simulink library "rewardLibrary"  (R2022b)
settings: Solver=VariableStepAuto  StartTime=0.0  StopTime=10.0  RelTol=1e-3
values from neighbouring files (symbols this model uses):
  accel_vec = (-4:0.5:4)'    [setUpModel.m]
  Ts = 0.1    [setUpMPC.m]
  TsRL = Ts    [setUpRLEnv.m]
  vel_vec = 0:2:20    [setUpModel.m]
undefined symbols (not defined in the file or in its folder): A, B, C, curvature1, D, D_default, DiscIntNeverNeededParam, E, F, gradbp1, k_sigmoid, steer_lim, t_gap, v_set, x_colpen, y_colpen, Z_colpen
libraries: simulink x379, $bdroot x2, mpcadaslib x1
(part 2 of 9)

== system rewardLibrary/Obs // Reward 6-1 ==
  xgap : Inport
  ygap : Inport  Port=2
  v_lead : Inport  Port=3
  v_ego : Inport  Port=4
  v_ref : Inport  Port=5
  e1 : Inport  Port=6
  e2 : Inport  Port=7
  e1dot : Inport  Port=8
  e2dot : Inport  Port=9
  accel : Inport  Port=10
  steer : Inport  Port=11
  collided : Inport  Port=12
  Abs : Abs  SaturateOnIntegerOverflow=off
  Compare To Constant : simulink/Logic and Bit Operations/Compare To Constant  relop=<=  const=6  OutDataTypeStr=boolean
  Gain1 : Gain  Gain=20
  Gain2 : Gain  Gain=1500
  Logical Operator1 : Logic  Operator=OR  AllPortsSameDT=off  OutDataTypeStr=boolean
  Subsystem : Subsystem
  Subsystem1 : Subsystem
  Subsystem2 : Subsystem
  Sum : Sum  Inputs=-++
  Terminator3 : Terminator
  obs : Outport  VectorParamsAs1DForOutWhenUnconnected=off
  Reward : Outport  Port=2  VectorParamsAs1DForOutWhenUnconnected=off
  isDone : Outport  Port=3  VectorParamsAs1DForOutWhenUnconnected=off
  tag scope: onTrack=global
  wires:
  Gain2/1 -> Sum/2
  Subsystem2/2(success) -> Gain2/1, Logical Operator1/2
  Subsystem2/1(fail) -> Logical Operator1/1, Gain1/1
  v_ego/1 -> Subsystem/1(v_ego), Subsystem2/1(v_ego)
  Logical Operator1/1 -> isDone/1
  accel/1 -> Subsystem1/5(accel)
  steer/1 -> Subsystem1/4(steer)
  Subsystem/2(v_err) -> Subsystem1/1(v_err)
  Subsystem1/1(reward) -> Sum/3
  ygap/1 -> Subsystem/9(ygap)
  v_ref/1 -> Subsystem/2(v_ref)
  collided/1 -> Terminator3/1
  Compare To Constant/1 -> [onTrack]
  Abs/1 -> Compare To Constant/1
  Gain1/1 -> Sum/1
  Sum/1 -> Reward/1
  e1dot/1 -> Subsystem/5(e1dot)
  Subsystem/1(obs) -> obs/1
  xgap/1 -> Subsystem/8(xgap)
  v_lead/1 -> Subsystem/7(v_lead)
  e2/1 -> Subsystem2/3(e2), Subsystem1/3(e2), Subsystem/4(e2)
  e1/1 -> Subsystem2/2(e1), Subsystem/3(e1), Subsystem1/2(e1), Abs/1
  e2dot/1 -> Subsystem/6(e2dot)

== system rewardLibrary/Obs // Reward 6-2 ==
  xgap : Inport
  ygap : Inport  Port=2
  v_lead : Inport  Port=3
  v_ego : Inport  Port=4
  v_ref : Inport  Port=5
  e1 : Inport  Port=6
  e2 : Inport  Port=7
  e1dot : Inport  Port=8
  e2dot : Inport  Port=9
  accel : Inport  Port=10
  steer : Inport  Port=11
  collided : Inport  Port=12
  A : Gain  Gain=1500
  Abs : Abs  SaturateOnIntegerOverflow=off
  B : Gain  Gain=2000
  Compare To Constant : simulink/Logic and Bit Operations/Compare To Constant  relop=<=  const=6  OutDataTypeStr=boolean
  E : Gain  Gain=2000
  Gain1 : Gain  Gain=20
  Logical Operator1 : Logic  Operator=OR  Inputs=3  AllPortsSameDT=off  OutDataTypeStr=boolean
  Overtaking : Subsystem
  Path following : Subsystem
  Subsystem : Subsystem
  Subsystem2 : Subsystem
  Sum : Sum  Inputs=--+++++
  Zone collision penalty : Lookup_n-D  BreakpointsForDimension1=y_colpen  BreakpointsForDimension2=x_colpen  Table=Z_colpen  ExtrapMethod=Clip  InternalRulePriority=Speed  RndMeth=Simplest
      settings: InputPortMap=u0,u1
      mask Display:
      | image("LookupTable.PNG")
      | port_label('input', 1, 'y')
      | port_label('input', 2, 'x')
      | port_label('output', 1, 'p_col')
  obs : Outport  VectorParamsAs1DForOutWhenUnconnected=off
  Reward : Outport  Port=2  VectorParamsAs1DForOutWhenUnconnected=off
  isDone : Outport  Port=3  VectorParamsAs1DForOutWhenUnconnected=off
  tag scope: onTrack=global, p_col=global
  wires:
  A/1 -> Sum/3
  Subsystem2/3(completeCourse) -> Logical Operator1/3, A/1
  Subsystem2/1(fail) -> Gain1/1, Logical Operator1/1
  v_ego/1 -> Subsystem/1(v_ego), Subsystem2/1(v_ego)
  Logical Operator1/1 -> isDone/1
  accel/1 -> Path following/5(accel)
  steer/1 -> Path following/4(steer)
  Subsystem/2(v_err) -> Path following/1(v_err)
  ygap/1 -> Zone collision penalty/1, Subsystem/9(ygap)
  v_ref/1 -> Subsystem/2(v_ref)
  collided/1 -> Subsystem2/5(collided)
  Compare To Constant/1 -> [onTrack]
  Abs/1 -> Compare To Constant/1
  Gain1/1 -> Sum/1
  Sum/1 -> Reward/1
  e1dot/1 -> Subsystem/5(e1dot)
  Subsystem/1(obs) -> obs/1
  xgap/1 -> Overtaking/2(G), Zone collision penalty/2, Subsystem2/4(xgap), Subsystem/8(xgap)
  v_lead/1 -> Subsystem/7(v_lead)
  e2/1 -> Subsystem2/3(e2), Path following/3(e2), Subsystem/4(e2)
  e1/1 -> Subsystem2/2(e1), Subsystem/3(e1), Path following/2(e1), Abs/1
  e2dot/1 -> Subsystem/6(e2dot)
  Path following/1(r_pf) -> Sum/5
  [ry2] -> Overtaking/1(ry)
  Subsystem2/4(overtakeSuccess) -> B/1
  B/1 -> Sum/4
  Overtaking/1(r_ot) -> Sum/6
  Subsystem2/2(failCollided) -> E/1, Logical Operator1/2
  E/1 -> Sum/2
  Zone collision penalty/1 -> Sum/7, [p_col]

== system rewardLibrary/Obs // Reward 6-3 ==
  xgap : Inport
  ygap : Inport  Port=2
  v_lead : Inport  Port=3
  v_ego : Inport  Port=4
  v_ref : Inport  Port=5
  e1 : Inport  Port=6
  e2 : Inport  Port=7
  e1dot : Inport  Port=8
  e2dot : Inport  Port=9
  accel : Inport  Port=10
  steer : Inport  Port=11
  collided : Inport  Port=12
  Abs : Abs  SaturateOnIntegerOverflow=off
  Compare To Constant : simulink/Logic and Bit Operations/Compare To Constant  relop=<=  const=6  OutDataTypeStr=boolean
  Gain1 : Gain  Gain=20
  Gain2 : Gain  Gain=1500
  Gain3 : Gain  Gain=100
  Logical Operator1 : Logic  Operator=OR  Inputs=3  AllPortsSameDT=off  OutDataTypeStr=boolean
  Subsystem : Subsystem
  Subsystem1 : Subsystem
  Subsystem2 : Subsystem
  Sum : Sum  Inputs=--++
  Terminator3 : Terminator
  obs : Outport  VectorParamsAs1DForOutWhenUnconnected=off
  Reward : Outport  Port=2  VectorParamsAs1DForOutWhenUnconnected=off
  isDone : Outport  Port=3  VectorParamsAs1DForOutWhenUnconnected=off
  tag scope: onTrack=global
  wires:
  Gain2/1 -> Sum/3
  Subsystem2/2(success) -> Gain2/1, Logical Operator1/2
  Subsystem2/1(fail) -> Gain1/1, Logical Operator1/1
  v_ego/1 -> Subsystem/1(v_ego), Subsystem2/1(v_ego)
  Logical Operator1/1 -> isDone/1
  accel/1 -> Subsystem1/5(accel)
  steer/1 -> Subsystem1/4(steer)
  Subsystem/2(v_err) -> Subsystem1/1(v_err)
  Subsystem1/1(reward) -> Sum/4
  ygap/1 -> Subsystem/9(ygap)
  v_ref/1 -> Subsystem/2(v_ref)
  collided/1 -> Terminator3/1
  Compare To Constant/1 -> [onTrack]
  Abs/1 -> Compare To Constant/1
  Gain1/1 -> Sum/1
  Sum/1 -> Reward/1
  e1dot/1 -> Subsystem/5(e1dot)
  Subsystem/1(obs) -> obs/1
  xgap/1 -> Subsystem/8(xgap)
  v_lead/1 -> Subsystem/7(v_lead)
  e2/1 -> Subsystem2/3(e2), Subsystem1/3(e2), Subsystem/4(e2)
  e1/1 -> Subsystem2/2(e1), Subsystem/3(e1), Subsystem1/2(e1), Abs/1
  e2dot/1 -> Subsystem/6(e2dot)
  Subsystem2/3(fail_spinTurn) -> Gain3/1, Logical Operator1/3
  Gain3/1 -> Sum/2

== system rewardLibrary/Obs // Reward 6-4 ==
  xgap : Inport
  ygap : Inport  Port=2
  v_lead : Inport  Port=3
  v_ego : Inport  Port=4
  v_ref : Inport  Port=5
  e1 : Inport  Port=6
  e2 : Inport  Port=7
  e1dot : Inport  Port=8
  e2dot : Inport  Port=9
  accel : Inport  Port=10
  steer : Inport  Port=11
  collided : Inport  Port=12
  Abs : Abs  SaturateOnIntegerOverflow=off
  Compare To Constant : simulink/Logic and Bit Operations/Compare To Constant  relop=<=  const=6  OutDataTypeStr=boolean
  Gain1 : Gain  Gain=20
  Gain2 : Gain  Gain=1500
  Logical Operator1 : Logic  Operator=OR  AllPortsSameDT=off  OutDataTypeStr=boolean
  Subsystem : Subsystem
  Subsystem1 : Subsystem
  Subsystem2 : Subsystem
  Sum : Sum  Inputs=-++
  Terminator3 : Terminator
  obs : Outport  VectorParamsAs1DForOutWhenUnconnected=off
  Reward : Outport  Port=2  VectorParamsAs1DForOutWhenUnconnected=off
  isDone : Outport  Port=3  VectorParamsAs1DForOutWhenUnconnected=off
  tag scope: onTrack=global
  wires:
  Gain2/1 -> Sum/2
  Subsystem2/2(success) -> Gain2/1, Logical Operator1/2
  Subsystem2/1(fail) -> Logical Operator1/1, Gain1/1
  v_ego/1 -> Subsystem/1(v_ego), Subsystem2/1(v_ego)
  Logical Operator1/1 -> isDone/1
  accel/1 -> Subsystem1/5(accel)
  steer/1 -> Subsystem1/4(steer)
  Subsystem/2(v_err) -> Subsystem1/1(v_err)
  ygap/1 -> Subsystem/9(ygap)
  v_ref/1 -> Subsystem/2(v_ref)
  collided/1 -> Terminator3/1
  Compare To Constant/1 -> [onTrack]
  Abs/1 -> Compare To Constant/1
  Gain1/1 -> Sum/1
  Sum/1 -> Reward/1
  e1dot/1 -> Subsystem/5(e1dot)
  Subsystem/1(obs) -> obs/1
  xgap/1 -> Subsystem/8(xgap)
  v_lead/1 -> Subsystem/7(v_lead)
  e2/1 -> Subsystem2/3(e2), Subsystem1/3(e2), Subsystem/4(e2)
  e1/1 -> Subsystem2/2(e1), Subsystem/3(e1), Subsystem1/2(e1), Abs/1
  e2dot/1 -> Subsystem/6(e2dot)
  Subsystem1/1(reward) -> Sum/3

== system rewardLibrary/Obs // Reward 6-5 ==
  xgap : Inport
  ygap : Inport  Port=2
  v_lead : Inport  Port=3
  v_ego : Inport  Port=4
  v_ref : Inport  Port=5
  e1 : Inport  Port=6
  e2 : Inport  Port=7
  e1dot : Inport  Port=8
  e2dot : Inport  Port=9
  accel : Inport  Port=10
  steer : Inport  Port=11
  collided : Inport  Port=12
  Abs : Abs  SaturateOnIntegerOverflow=off
  Compare To Constant : simulink/Logic and Bit Operations/Compare To Constant  relop=<=  const=6  OutDataTypeStr=boolean
  Gain1 : Gain  Gain=20
  Gain2 : Gain  Gain=1500
  Logical Operator1 : Logic  Operator=OR  AllPortsSameDT=off  OutDataTypeStr=boolean
  Subsystem : Subsystem
  Subsystem1 : Subsystem
  Subsystem2 : Subsystem
  Sum : Sum  Inputs=-++
  Terminator3 : Terminator
  obs : Outport  VectorParamsAs1DForOutWhenUnconnected=off
  Reward : Outport  Port=2  VectorParamsAs1DForOutWhenUnconnected=off
  isDone : Outport  Port=3  VectorParamsAs1DForOutWhenUnconnected=off
  tag scope: onTrack=global
  wires:
  Gain2/1 -> Sum/2
  Subsystem2/2(success) -> Gain2/1, Logical Operator1/2
  Subsystem2/1(fail) -> Logical Operator1/1, Gain1/1
  v_ego/1 -> Subsystem/1(v_ego), Subsystem2/1(v_ego)
  Logical Operator1/1 -> isDone/1
  accel/1 -> Subsystem1/5(accel)
  steer/1 -> Subsystem1/4(steer)
  Subsystem/2(v_err) -> Subsystem1/1(v_err)
  ygap/1 -> Subsystem/9(ygap)
  v_ref/1 -> Subsystem/2(v_ref)
  collided/1 -> Terminator3/1
  Compare To Constant/1 -> [onTrack]
  Abs/1 -> Compare To Constant/1
  Gain1/1 -> Sum/1
  Sum/1 -> Reward/1
  e1dot/1 -> Subsystem/5(e1dot)
  Subsystem/1(obs) -> obs/1
  xgap/1 -> Subsystem/8(xgap)
  v_lead/1 -> Subsystem/7(v_lead)
  e2/1 -> Subsystem2/3(e2), Subsystem1/3(e2), Subsystem/4(e2)
  e1/1 -> Subsystem2/2(e1), Subsystem/3(e1), Subsystem1/2(e1), Abs/1
  e2dot/1 -> Subsystem/6(e2dot)
  Subsystem1/1(reward) -> Sum/3

== system rewardLibrary/Obs // Reward 7-1 ==
  xgap : Inport
  ygap : Inport  Port=2
  v_lead : Inport  Port=3
  v_ego : Inport  Port=4
  v_ref : Inport  Port=5
  e1 : Inport  Port=6
  e2 : Inport  Port=7
  e1dot : Inport  Port=8
  e2dot : Inport  Port=9
  accel : Inport  Port=10
  steer : Inport  Port=11
  collided : Inport  Port=12
  Abs : Abs  SaturateOnIntegerOverflow=off
  Compare To Constant : simulink/Logic and Bit Operations/Compare To Constant  relop=<=  const=6  OutDataTypeStr=boolean
  Gain1 : Gain  Gain=20
  Gain2 : Gain  Gain=1500
  Gain3 : Gain  Gain=B
  Logical Operator1 : Logic  Operator=OR  AllPortsSameDT=off  OutDataTypeStr=boolean
  Overtaking : Subsystem
  Path following : Subsystem
  Subsystem : Subsystem
  Subsystem2 : Subsystem
  Sum : Sum  Inputs=-++++
  Terminator3 : Terminator
  obs : Outport  VectorParamsAs1DForOutWhenUnconnected=off
  Reward : Outport  Port=2  VectorParamsAs1DForOutWhenUnconnected=off
  isDone : Outport  Port=3  VectorParamsAs1DForOutWhenUnconnected=off
  tag scope: onTrack=global
  wires:
  Gain2/1 -> Sum/2
  Subsystem2/2(completeCourse) -> Gain2/1, Logical Operator1/2
  Subsystem2/1(fail) -> Logical Operator1/1, Gain1/1
  v_ego/1 -> Subsystem/1(v_ego), Subsystem2/1(v_ego)
  Logical Operator1/1 -> isDone/1
  accel/1 -> Path following/5(accel)
  steer/1 -> Path following/4(steer)
  Subsystem/2(v_err) -> Path following/1(v_err)
  ygap/1 -> Subsystem/9(ygap)
  v_ref/1 -> Subsystem/2(v_ref)
  collided/1 -> Terminator3/1
  Compare To Constant/1 -> [onTrack]
  Abs/1 -> Compare To Constant/1
  Gain1/1 -> Sum/1
  Sum/1 -> Reward/1
  e1dot/1 -> Subsystem/5(e1dot)
  Subsystem/1(obs) -> obs/1
  xgap/1 -> Overtaking/2(G), Subsystem2/4(xgap), Subsystem/8(xgap)
  v_lead/1 -> Subsystem/7(v_lead)
  e2/1 -> Subsystem2/3(e2), Path following/3(e2), Subsystem/4(e2)
  e1/1 -> Subsystem2/2(e1), Subsystem/3(e1), Path following/2(e1), Abs/1
  e2dot/1 -> Subsystem/6(e2dot)
  Path following/1(r_pf) -> Sum/4
  [ry2] -> Overtaking/1(ry)
  Subsystem2/3(overtakeSuccess) -> Gain3/1
  Gain3/1 -> Sum/3
  Overtaking/1(r_ot) -> Sum/5

== system rewardLibrary/Obs // Reward 7-2 ==
  xgap : Inport
  ygap : Inport  Port=2
  v_lead : Inport  Port=3
  v_ego : Inport  Port=4
  v_ref : Inport  Port=5
  e1 : Inport  Port=6
  e2 : Inport  Port=7
  e1dot : Inport  Port=8
  e2dot : Inport  Port=9
  accel : Inport  Port=10
  steer : Inport  Port=11
  collided : Inport  Port=12
  Abs : Abs  SaturateOnIntegerOverflow=off
  Compare To Constant : simulink/Logic and Bit Operations/Compare To Constant  relop=<=  const=6  OutDataTypeStr=boolean
  Gain1 : Gain  Gain=20
  Gain2 : Gain  Gain=A
  Gain3 : Gain  Gain=B
  Logical Operator1 : Logic  Operator=OR  AllPortsSameDT=off  OutDataTypeStr=boolean
  Overtaking : Subsystem
  Path following : Subsystem
  Subsystem : Subsystem
  Subsystem2 : Subsystem
  Sum : Sum  Inputs=-++++
  Terminator3 : Terminator
  obs : Outport  VectorParamsAs1DForOutWhenUnconnected=off
  Reward : Outport  Port=2  VectorParamsAs1DForOutWhenUnconnected=off
  isDone : Outport  Port=3  VectorParamsAs1DForOutWhenUnconnected=off
  tag scope: onTrack=global
  wires:
  Gain2/1 -> Sum/2
  Subsystem2/2(completeCourse) -> Gain2/1, Logical Operator1/2
  Subsystem2/1(fail) -> Logical Operator1/1, Gain1/1
  v_ego/1 -> Subsystem/1(v_ego), Subsystem2/1(v_ego)
  Logical Operator1/1 -> isDone/1
  accel/1 -> Path following/5(accel)
  steer/1 -> Path following/4(steer)
  Subsystem/2(v_err) -> Path following/1(v_err)
  ygap/1 -> Subsystem/9(ygap)
  v_ref/1 -> Subsystem/2(v_ref)
  collided/1 -> Terminator3/1
  Compare To Constant/1 -> [onTrack]
  Abs/1 -> Compare To Constant/1
  Gain1/1 -> Sum/1
  Sum/1 -> Reward/1
  e1dot/1 -> Subsystem/5(e1dot)
  Subsystem/1(obs) -> obs/1
  xgap/1 -> Overtaking/2(G), Subsystem2/4(xgap), Subsystem/8(xgap)
  v_lead/1 -> Subsystem/7(v_lead)
  e2/1 -> Subsystem2/3(e2), Path following/3(e2), Subsystem/4(e2)
  e1/1 -> Subsystem2/2(e1), Subsystem/3(e1), Path following/2(e1), Abs/1
  e2dot/1 -> Subsystem/6(e2dot)
  Path following/1(r_pf) -> Sum/4
  [ry2] -> Overtaking/1(ry)
  Subsystem2/3(overtakeSuccess) -> Gain3/1
  Gain3/1 -> Sum/3
  Overtaking/1(r_ot) -> Sum/5

== system rewardLibrary/Obs // Reward 8-1 ==
  xgap : Inport
  ygap : Inport  Port=2
  v_lead : Inport  Port=3
  v_ego : Inport  Port=4
  v_ref : Inport  Port=5
  e1 : Inport  Port=6
  e2 : Inport  Port=7
  e1dot : Inport  Port=8
  e2dot : Inport  Port=9
  accel : Inport  Port=10
  steer : Inport  Port=11
  collided : Inport  Port=12
  Abs : Abs  SaturateOnIntegerOverflow=off
  Compare To Constant : simulink/Logic and Bit Operations/Compare To Constant  relop=<=  const=6  OutDataTypeStr=boolean
  Gain1 : Gain  Gain=20
  Gain2 : Gain  Gain=1500
  Gain3 : Gain  Gain=B
  Gain4 : Gain  Gain=3000
  Logical Operator1 : Logic  Operator=OR  Inputs=3  AllPortsSameDT=off  OutDataTypeStr=boolean
  Overtaking : Subsystem
  Path following : Subsystem
  Subsystem : Subsystem
  Subsystem2 : Subsystem
  Sum : Sum  Inputs=--++++
  obs : Outport  VectorParamsAs1DForOutWhenUnconnected=off
  Reward : Outport  Port=2  VectorParamsAs1DForOutWhenUnconnected=off
  isDone : Outport  Port=3  VectorParamsAs1DForOutWhenUnconnected=off
  tag scope: onTrack=global
  wires:
  Gain2/1 -> Sum/3
  Subsystem2/3(completeCourse) -> Logical Operator1/3, Gain2/1
  Subsystem2/1(fail) -> Gain1/1, Logical Operator1/1
  v_ego/1 -> Subsystem/1(v_ego), Subsystem2/1(v_ego)
  Logical Operator1/1 -> isDone/1
  accel/1 -> Path following/5(accel)
  steer/1 -> Path following/4(steer)
  Subsystem/2(v_err) -> Path following/1(v_err)
  ygap/1 -> Subsystem/9(ygap)
  v_ref/1 -> Subsystem/2(v_ref)
  collided/1 -> Subsystem2/5(collided)
  Compare To Constant/1 -> [onTrack]
  Abs/1 -> Compare To Constant/1
  Gain1/1 -> Sum/1
  Sum/1 -> Reward/1
  e1dot/1 -> Subsystem/5(e1dot)
  Subsystem/1(obs) -> obs/1
  xgap/1 -> Overtaking/2(G), Subsystem2/4(xgap), Subsystem/8(xgap)
  v_lead/1 -> Subsystem/7(v_lead)
  e2/1 -> Subsystem2/3(e2), Path following/3(e2), Subsystem/4(e2)
  e1/1 -> Subsystem2/2(e1), Subsystem/3(e1), Path following/2(e1), Abs/1
  e2dot/1 -> Subsystem/6(e2dot)
  Path following/1(r_pf) -> Sum/5
  [ry2] -> Overtaking/1(ry)
  Subsystem2/4(overtakeSuccess) -> Gain3/1
  Gain3/1 -> Sum/4
  Overtaking/1(r_ot) -> Sum/6
  Subsystem2/2(failCollided) -> Gain4/1, Logical Operator1/2
  Gain4/1 -> Sum/2

== system rewardLibrary/Obs // Reward 8-10 ==
  xgap : Inport
  ygap : Inport  Port=2
  v_lead : Inport  Port=3
  v_ego : Inport  Port=4
  v_ref : Inport  Port=5
  e1 : Inport  Port=6
  e2 : Inport  Port=7
  e1dot : Inport  Port=8
  e2dot : Inport  Port=9
  accel : Inport  Port=10
  steer : Inport  Port=11
  collided : Inport  Port=12
  A : Gain  Gain=0
  Abs : Abs  SaturateOnIntegerOverflow=off
  B : Gain  Gain=2000
  Compare To Constant : simulink/Logic and Bit Operations/Compare To Constant  relop=<=  const=6  OutDataTypeStr=boolean
  E : Gain  Gain=2000
  Gain1 : Gain  Gain=20
  Logical Operator1 : Logic  Operator=OR  Inputs=3  AllPortsSameDT=off  OutDataTypeStr=boolean
  Overtaking : Subsystem
  Path following : Subsystem
  Subsystem : Subsystem
  Subsystem2 : Subsystem
  Sum : Sum  Inputs=--+++++
  Zone collision penalty : Lookup_n-D  BreakpointsForDimension1=y_colpen  BreakpointsForDimension2=x_colpen  Table=Z_colpen  ExtrapMethod=Clip  InternalRulePriority=Speed  RndMeth=Simplest
      settings: InputPortMap=u0,u1
      mask Display:
      | image("LookupTable.PNG")
      | port_label('input', 1, 'y')
      | port_label('input', 2, 'x')
      | port_label('output', 1, 'p_col')
  obs : Outport  VectorParamsAs1DForOutWhenUnconnected=off
  Reward : Outport  Port=2  VectorParamsAs1DForOutWhenUnconnected=off
  isDone : Outport  Port=3  VectorParamsAs1DForOutWhenUnconnected=off
  tag scope: onTrack=global, p_col=global
  wires:
  Zone collision penalty/1 -> [p_col], Sum/7
  E/1 -> Sum/2
  Subsystem2/2(failCollided) -> Logical Operator1/2, E/1
  Overtaking/1(r_ot) -> Sum/6
  B/1 -> Sum/4
  Subsystem2/4(overtakeSuccess) -> B/1
  [ry2] -> Overtaking/1(ry)
  Path following/1(r_pf) -> Sum/5
  e2dot/1 -> Subsystem/6(e2dot)
  e1/1 -> Abs/1, Path following/2(e1), Subsystem/3(e1), Subsystem2/2(e1)
  e2/1 -> Subsystem/4(e2), Path following/3(e2), Subsystem2/3(e2)
  v_lead/1 -> Subsystem/7(v_lead)
  xgap/1 -> Subsystem/8(xgap), Subsystem2/4(xgap), Zone collision penalty/2, Overtaking/2(G)
  Subsystem/1(obs) -> obs/1
  e1dot/1 -> Subsystem/5(e1dot)
  Sum/1 -> Reward/1
  Gain1/1 -> Sum/1
  Abs/1 -> Compare To Constant/1
  Compare To Constant/1 -> [onTrack]
  collided/1 -> Subsystem2/5(collided)
  v_ref/1 -> Subsystem/2(v_ref)
  ygap/1 -> Subsystem/9(ygap), Zone collision penalty/1
  Subsystem/2(v_err) -> Path following/1(v_err)
  steer/1 -> Path following/4(steer)
  accel/1 -> Path following/5(accel)
  Logical Operator1/1 -> isDone/1
  v_ego/1 -> Subsystem2/1(v_ego), Subsystem/1(v_ego)
  Subsystem2/1(fail) -> Logical Operator1/1, Gain1/1
  Subsystem2/3(completeCourse) -> A/1, Logical Operator1/3
  A/1 -> Sum/3

== system rewardLibrary/Obs // Reward 8-11 ==
  xgap : Inport
  ygap : Inport  Port=2
  v_lead : Inport  Port=3
  v_ego : Inport  Port=4
  v_ref : Inport  Port=5
  e1 : Inport  Port=6
  e2 : Inport  Port=7
  e1dot : Inport  Port=8
  e2dot : Inport  Port=9
  accel : Inport  Port=10
  steer : Inport  Port=11
  collided : Inport  Port=12
  A : Gain  Gain=0
  Abs : Abs  SaturateOnIntegerOverflow=off
  B : Gain  Gain=2000
  Compare To Constant : simulink/Logic and Bit Operations/Compare To Constant  relop=<=  const=6  OutDataTypeStr=boolean
  E : Gain  Gain=2000
  Gain1 : Gain  Gain=20
  Logical Operator1 : Logic  Operator=OR  Inputs=3  AllPortsSameDT=off  OutDataTypeStr=boolean
  Overtaking : Subsystem
  Path following : Subsystem
  Subsystem : Subsystem
  Subsystem2 : Subsystem
  Sum : Sum  Inputs=--+++++
  Zone collision penalty : Lookup_n-D  BreakpointsForDimension1=y_colpen  BreakpointsForDimension2=x_colpen  Table=Z_colpen  ExtrapMethod=Clip  InternalRulePriority=Speed  RndMeth=Simplest
      settings: InputPortMap=u0,u1
      mask Display:
      | image("LookupTable.PNG")
      | port_label('input', 1, 'y')
      | port_label('input', 2, 'x')
      | port_label('output', 1, 'p_col')
  obs : Outport  VectorParamsAs1DForOutWhenUnconnected=off
  Reward : Outport  Port=2  VectorParamsAs1DForOutWhenUnconnected=off
  isDone : Outport  Port=3  VectorParamsAs1DForOutWhenUnconnected=off
  tag scope: onTrack=global, p_col=global
  wires:
  Zone collision penalty/1 -> [p_col], Sum/7
  E/1 -> Sum/2
  Subsystem2/2(failCollided) -> Logical Operator1/2, E/1
  Overtaking/1(r_ot) -> Sum/6
  B/1 -> Sum/4
  Subsystem2/4(overtakeSuccess) -> B/1
  [ry2] -> Overtaking/1(ry)
  Path following/1(r_pf) -> Sum/5
  e2dot/1 -> Subsystem/6(e2dot)
  e1/1 -> Abs/1, Path following/2(e1), Subsystem/3(e1), Subsystem2/2(e1)
  e2/1 -> Subsystem/4(e2), Path following/3(e2), Subsystem2/3(e2)
  v_lead/1 -> Subsystem/7(v_lead)
  xgap/1 -> Subsystem/8(xgap), Subsystem2/4(xgap), Zone collision penalty/2, Overtaking/2(G)
  Subsystem/1(obs) -> obs/1
  e1dot/1 -> Subsystem/5(e1dot)
  Sum/1 -> Reward/1
  Gain1/1 -> Sum/1
  Abs/1 -> Compare To Constant/1
  Compare To Constant/1 -> [onTrack]
  collided/1 -> Subsystem2/5(collided)
  v_ref/1 -> Subsystem/2(v_ref)
  ygap/1 -> Subsystem/9(ygap), Zone collision penalty/1
  Subsystem/2(v_err) -> Path following/1(v_err)
  steer/1 -> Path following/4(steer)
  accel/1 -> Path following/5(accel)
  Logical Operator1/1 -> isDone/1
  v_ego/1 -> Subsystem2/1(v_ego), Subsystem/1(v_ego)
  Subsystem2/1(fail) -> Logical Operator1/1, Gain1/1
  Subsystem2/3(completeCourse) -> A/1, Logical Operator1/3
  A/1 -> Sum/3

== system rewardLibrary/Obs // Reward 8-12 ==
  xgap : Inport
  ygap : Inport  Port=2
  v_lead : Inport  Port=3
  v_ego : Inport  Port=4
  v_ref : Inport  Port=5
  e1 : Inport  Port=6
  e2 : Inport  Port=7
  e1dot : Inport  Port=8
  e2dot : Inport  Port=9
  accel : Inport  Port=10
  steer : Inport  Port=11
  collided : Inport  Port=12
  A : Gain  Gain=0
  Abs : Abs  SaturateOnIntegerOverflow=off
  B : Gain  Gain=2000
  Compare To Constant : simulink/Logic and Bit Operations/Compare To Constant  relop=<=  const=6  OutDataTypeStr=boolean
  E : Gain  Gain=2000
  Gain1 : Gain  Gain=20
  Logical Operator1 : Logic  Operator=OR  Inputs=3  AllPortsSameDT=off  OutDataTypeStr=boolean
  Overtaking : Subsystem
  Path following : Subsystem
  Subsystem : Subsystem
  Subsystem2 : Subsystem
  Sum : Sum  Inputs=--+++++
  Zone collision penalty : Lookup_n-D  BreakpointsForDimension1=y_colpen  BreakpointsForDimension2=x_colpen  Table=Z_colpen  ExtrapMethod=Clip  InternalRulePriority=Speed  RndMeth=Simplest
      settings: InputPortMap=u0,u1
      mask Display:
      | image("LookupTable.PNG")
      | port_label('input', 1, 'y')
      | port_label('input', 2, 'x')
      | port_label('output', 1, 'p_col')
  obs : Outport  VectorParamsAs1DForOutWhenUnconnected=off
  Reward : Outport  Port=2  VectorParamsAs1DForOutWhenUnconnected=off
  isDone : Outport  Port=3  VectorParamsAs1DForOutWhenUnconnected=off
  tag scope: onTrack=global, p_col=global
  wires:
  Zone collision penalty/1 -> [p_col], Sum/7
  E/1 -> Sum/2
  Subsystem2/2(failCollided) -> Logical Operator1/2, E/1
  Overtaking/1(r_ot) -> Sum/6
  B/1 -> Sum/4
  Subsystem2/4(overtakeSuccess) -> B/1
  [ry2] -> Overtaking/1(ry)
  Path following/1(r_pf) -> Sum/5
  e2dot/1 -> Subsystem/6(e2dot)
  e1/1 -> Abs/1, Path following/2(e1), Subsystem/3(e1), Subsystem2/2(e1)
  e2/1 -> Subsystem/4(e2), Path following/3(e2), Subsystem2/3(e2)
  v_lead/1 -> Subsystem/7(v_lead)
  xgap/1 -> Subsystem/8(xgap), Subsystem2/4(xgap), Zone collision penalty/2, Overtaking/2(G)
  Subsystem/1(obs) -> obs/1
  e1dot/1 -> Subsystem/5(e1dot)
  Sum/1 -> Reward/1
  Gain1/1 -> Sum/1
  Abs/1 -> Compare To Constant/1
  Compare To Constant/1 -> [onTrack]
  collided/1 -> Subsystem2/5(collided)
  v_ref/1 -> Subsystem/2(v_ref)
  ygap/1 -> Subsystem/9(ygap), Zone collision penalty/1
  Subsystem/2(v_err) -> Path following/1(v_err)
  steer/1 -> Path following/4(steer)
  accel/1 -> Path following/5(accel)
  Logical Operator1/1 -> isDone/1
  v_ego/1 -> Subsystem2/1(v_ego), Subsystem/1(v_ego)
  Subsystem2/1(fail) -> Logical Operator1/1, Gain1/1
  Subsystem2/3(completeCourse) -> A/1, Logical Operator1/3
  A/1 -> Sum/3

== system rewardLibrary/Obs // Reward 8-13 ==
  xgap : Inport
  ygap : Inport  Port=2
  v_lead : Inport  Port=3
  v_ego : Inport  Port=4
  v_ref : Inport  Port=5
  e1 : Inport  Port=6
  e2 : Inport  Port=7
  e1dot : Inport  Port=8
  e2dot : Inport  Port=9
  accel : Inport  Port=10
  steer : Inport  Port=11
  collided : Inport  Port=12
  A : Gain  Gain=0
  Abs : Abs  SaturateOnIntegerOverflow=off
  B : Gain  Gain=2000
  Compare To Constant : simulink/Logic and Bit Operations/Compare To Constant  relop=<=  const=6  OutDataTypeStr=boolean
  E : Gain  Gain=2000
  Gain1 : Gain  Gain=20
  Logical Operator1 : Logic  Operator=OR  Inputs=3  AllPortsSameDT=off  OutDataTypeStr=boolean
  Overtaking : Subsystem
  Path following : Subsystem
  Subsystem : Subsystem
  Subsystem2 : Subsystem
  Sum : Sum  Inputs=--+++++
  Zone collision penalty : Lookup_n-D  BreakpointsForDimension1=y_colpen  BreakpointsForDimension2=x_colpen  Table=Z_colpen  ExtrapMethod=Clip  InternalRulePriority=Speed  RndMeth=Simplest
      settings: InputPortMap=u0,u1
      mask Display:
      | image("LookupTable.PNG")
      | port_label('input', 1, 'y')
      | port_label('input', 2, 'x')
      | port_label('output', 1, 'p_col')
  obs : Outport  VectorParamsAs1DForOutWhenUnconnected=off
  Reward : Outport  Port=2  VectorParamsAs1DForOutWhenUnconnected=off
  isDone : Outport  Port=3  VectorParamsAs1DForOutWhenUnconnected=off
  tag scope: onTrack=global, p_col=global
  wires:
  Zone collision penalty/1 -> [p_col], Sum/7
  E/1 -> Sum/2
  Subsystem2/2(failCollided) -> Logical Operator1/2, E/1
  Overtaking/1(r_ot) -> Sum/6
  B/1 -> Sum/4
  Subsystem2/4(overtakeSuccess) -> B/1
  [ry2] -> Overtaking/1(ry)
  Path following/1(r_pf) -> Sum/5
  e2dot/1 -> Subsystem/6(e2dot)
  e1/1 -> Abs/1, Path following/2(e1), Subsystem/3(e1), Subsystem2/2(e1)
  e2/1 -> Subsystem/4(e2), Path following/3(e2), Subsystem2/3(e2)
  v_lead/1 -> Subsystem/7(v_lead)
  xgap/1 -> Subsystem/8(xgap), Subsystem2/4(xgap), Zone collision penalty/2, Overtaking/2(G)
  Subsystem/1(obs) -> obs/1
  e1dot/1 -> Subsystem/5(e1dot)
  Sum/1 -> Reward/1
  Gain1/1 -> Sum/1
  Abs/1 -> Compare To Constant/1
  Compare To Constant/1 -> [onTrack]
  collided/1 -> Subsystem2/5(collided)
  v_ref/1 -> Subsystem/2(v_ref)
  ygap/1 -> Subsystem/9(ygap), Zone collision penalty/1
  Subsystem/2(v_err) -> Path following/1(v_err)
  steer/1 -> Path following/4(steer)
  accel/1 -> Path following/5(accel)
  Logical Operator1/1 -> isDone/1
  v_ego/1 -> Subsystem2/1(v_ego), Subsystem/1(v_ego)
  Subsystem2/1(fail) -> Logical Operator1/1, Gain1/1
  Subsystem2/3(completeCourse) -> A/1, Logical Operator1/3
  A/1 -> Sum/3

== system rewardLibrary/Obs // Reward 8-14 ==
  xgap : Inport
  ygap : Inport  Port=2
  v_lead : Inport  Port=3
  v_ego : Inport  Port=4
  v_ref : Inport  Port=5
  e1 : Inport  Port=6
  e2 : Inport  Port=7
  e1dot : Inport  Port=8
  e2dot : Inport  Port=9
  accel : Inport  Port=10
  steer : Inport  Port=11
  collided : Inport  Port=12
  A : Gain  Gain=0
  Abs : Abs  SaturateOnIntegerOverflow=off
  B : Gain  Gain=2000
  Compare To Constant : simulink/Logic and Bit Operations/Compare To Constant  relop=<=  const=6  OutDataTypeStr=boolean
  E : Gain  Gain=2000
  Gain1 : Gain  Gain=20
  Logical Operator1 : Logic  Operator=OR  Inputs=3  AllPortsSameDT=off  OutDataTypeStr=boolean
  Overtaking : Subsystem
  Path following : Subsystem
  Subsystem : Subsystem
  Subsystem2 : Subsystem
  Sum : Sum  Inputs=--++
  Sum1 : Sum  Inputs=+++
  Sum2 : Sum
  Zone collision penalty : Lookup_n-D  BreakpointsForDimension1=y_colpen  BreakpointsForDimension2=x_colpen  Table=Z_colpen  ExtrapMethod=Clip  InternalRulePriority=Speed  RndMeth=Simplest
      settings: InputPortMap=u0,u1
      mask Display:
      | image("LookupTable.PNG")
      | port_label('input', 1, 'y')
      | port_label('input', 2, 'x')
      | port_label('output', 1, 'p_col')
  obs : Outport  VectorParamsAs1DForOutWhenUnconnected=off
  Reward : Outport  Port=2  VectorParamsAs1DForOutWhenUnconnected=off
  isDone : Outport  Port=3  VectorParamsAs1DForOutWhenUnconnected=off
  tag scope: onTrack=global, p_col=global
  wires:
  Zone collision penalty/1 -> Sum1/3, [p_col]
  E/1 -> Sum/2
  Subsystem2/2(failCollided) -> Logical Operator1/2, E/1
  Overtaking/1(r_ot) -> Sum1/2
  B/1 -> Sum/4
  Subsystem2/4(overtakeSuccess) -> B/1
  [ry2] -> Overtaking/1(ry)
  Path following/1(r_pf) -> Sum1/1
  e2dot/1 -> Subsystem/6(e2dot)
  e1/1 -> Abs/1, Path following/2(e1), Subsystem/3(e1), Subsystem2/2(e1)
  e2/1 -> Subsystem/4(e2), Path following/3(e2), Subsystem2/3(e2)
  v_lead/1 -> Subsystem/7(v_lead)
  xgap/1 -> Subsystem/8(xgap), Subsystem2/4(xgap), Zone collision penalty/2, Overtaking/2(G)
  Subsystem/1(obs) -> obs/1
  e1dot/1 -> Subsystem/5(e1dot)
  Gain1/1 -> Sum/1
  Abs/1 -> Compare To Constant/1
  Compare To Constant/1 -> [onTrack]
  collided/1 -> Subsystem2/5(collided)
  v_ref/1 -> Subsystem/2(v_ref)
  ygap/1 -> Subsystem/9(ygap), Zone collision penalty/1
  Subsystem/2(v_err) -> Path following/1(v_err)
  steer/1 -> Path following/4(steer)
  accel/1 -> Path following/5(accel)
  Logical Operator1/1 -> isDone/1
  v_ego/1 -> Subsystem2/1(v_ego), Subsystem/1(v_ego)
  Subsystem2/1(fail) -> Logical Operator1/1, Gain1/1
  Subsystem2/3(completeCourse) -> A/1, Logical Operator1/3
  A/1 -> Sum/3
  Sum2/1 -> Reward/1
  Sum/1 -> Sum2/1
  Sum1/1 -> Sum2/2

== system rewardLibrary/Obs // Reward 8-15 ==
  xgap : Inport
  ygap : Inport  Port=2
  v_lead : Inport  Port=3
  v_ego : Inport  Port=4
  v_ref : Inport  Port=5
  e1 : Inport  Port=6
  e2 : Inport  Port=7
  e1dot : Inport  Port=8
  e2dot : Inport  Port=9
  accel : Inport  Port=10
  steer : Inport  Port=11
  collided : Inport  Port=12
  A : Gain  Gain=0
  Abs : Abs  SaturateOnIntegerOverflow=off
  B : Gain  Gain=2000
  Compare To Constant : simulink/Logic and Bit Operations/Compare To Constant  relop=<=  const=6  OutDataTypeStr=boolean
  E : Gain  Gain=2000
  Gain1 : Gain  Gain=20
  Logical Operator1 : Logic  Operator=OR  Inputs=3  AllPortsSameDT=off  OutDataTypeStr=boolean
  Overtaking : Subsystem
  Path following : Subsystem
  Subsystem : Subsystem
  Subsystem2 : Subsystem
  Sum : Sum  Inputs=--++
  Sum1 : Sum  Inputs=+++
  Sum2 : Sum
  Zone collision penalty : Lookup_n-D  BreakpointsForDimension1=y_colpen  BreakpointsForDimension2=x_colpen  Table=Z_colpen  ExtrapMethod=Clip  InternalRulePriority=Speed  RndMeth=Simplest
      settings: InputPortMap=u0,u1
      mask Display:
      | image("LookupTable.PNG")
      | port_label('input', 1, 'y')
      | port_label('input', 2, 'x')
      | port_label('output', 1, 'p_col')
  obs : Outport  VectorParamsAs1DForOutWhenUnconnected=off
  Reward : Outport  Port=2  VectorParamsAs1DForOutWhenUnconnected=off
  isDone : Outport  Port=3  VectorParamsAs1DForOutWhenUnconnected=off
  tag scope: onTrack=global, p_col=global
  wires:
  Zone collision penalty/1 -> Sum1/3, [p_col]
  E/1 -> Sum/2
  Subsystem2/2(failCollided) -> Logical Operator1/2, E/1
  Overtaking/1(r_ot) -> Sum1/2
  B/1 -> Sum/4
  Subsystem2/4(overtakeSuccess) -> B/1
  [ry2] -> Overtaking/1(ry)
  Path following/1(r_pf) -> Sum1/1
  e2dot/1 -> Subsystem/6(e2dot)
  e1/1 -> Abs/1, Path following/2(e1), Subsystem/3(e1), Subsystem2/2(e1)
  e2/1 -> Subsystem/4(e2), Path following/3(e2), Subsystem2/3(e2)
  v_lead/1 -> Subsystem/7(v_lead)
  xgap/1 -> Subsystem/8(xgap), Subsystem2/4(xgap), Zone collision penalty/2, Overtaking/2(G)
  Subsystem/1(obs) -> obs/1
  e1dot/1 -> Subsystem/5(e1dot)
  Gain1/1 -> Sum/1
  Abs/1 -> Compare To Constant/1
  Compare To Constant/1 -> [onTrack]
  collided/1 -> Subsystem2/5(collided)
  v_ref/1 -> Subsystem/2(v_ref)
  ygap/1 -> Subsystem/9(ygap), Zone collision penalty/1
  Subsystem/2(v_err) -> Path following/1(v_err)
  steer/1 -> Path following/4(steer)
  accel/1 -> Path following/5(accel)
  Logical Operator1/1 -> isDone/1
  v_ego/1 -> Subsystem2/1(v_ego), Subsystem/1(v_ego)
  Subsystem2/1(fail) -> Logical Operator1/1, Gain1/1
  Subsystem2/3(completeCourse) -> A/1, Logical Operator1/3
  A/1 -> Sum/3
  Sum2/1 -> Reward/1
  Sum/1 -> Sum2/1
  Sum1/1 -> Sum2/2

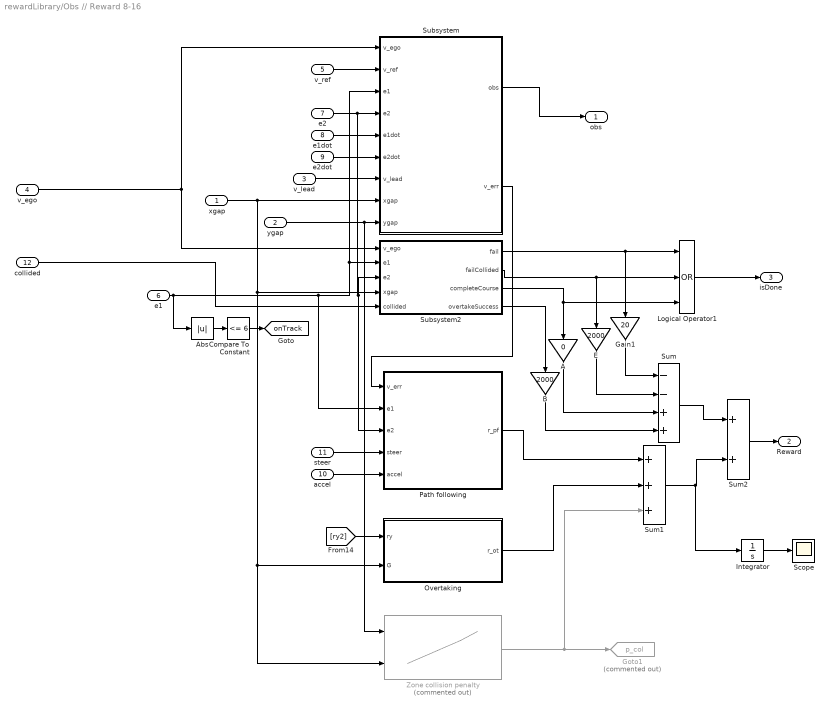
== system rewardLibrary/Obs // Reward 8-16 ==
  xgap : Inport
  ygap : Inport  Port=2
  v_lead : Inport  Port=3
  v_ego : Inport  Port=4
  v_ref : Inport  Port=5
  e1 : Inport  Port=6
  e2 : Inport  Port=7
  e1dot : Inport  Port=8
  e2dot : Inport  Port=9
  accel : Inport  Port=10
  steer : Inport  Port=11
  collided : Inport  Port=12
  A : Gain  Gain=0
  Abs : Abs  SaturateOnIntegerOverflow=off
  B : Gain  Gain=2000
  Compare To Constant : simulink/Logic and Bit Operations/Compare To Constant  relop=<=  const=6  OutDataTypeStr=boolean
  E : Gain  Gain=2000
  Gain1 : Gain  Gain=20
  Goto1 : Goto  Commented=on  GotoTag=p_col  TagVisibility=global
  Integrator : Integrator
  Logical Operator1 : Logic  Operator=OR  Inputs=3  AllPortsSameDT=off  OutDataTypeStr=boolean
  Overtaking : Subsystem
  Path following : Subsystem
  Scope : Scope
  Subsystem : Subsystem
  Subsystem2 : Subsystem
  Sum : Sum  Inputs=--++
  Sum1 : Sum  Inputs=+++
  Sum2 : Sum
  Zone collision penalty : Lookup_n-D  Commented=on  BreakpointsForDimension1=y_colpen  BreakpointsForDimension2=x_colpen  Table=Z_colpen  ExtrapMethod=Clip  InternalRulePriority=Speed  RndMeth=Simplest
      settings: InputPortMap=u0,u1
      mask Display:
      | image("LookupTable.PNG")
      | port_label('input', 1, 'y')
      | port_label('input', 2, 'x')
      | port_label('output', 1, 'p_col')
  obs : Outport  VectorParamsAs1DForOutWhenUnconnected=off
  Reward : Outport  Port=2  VectorParamsAs1DForOutWhenUnconnected=off
  isDone : Outport  Port=3  VectorParamsAs1DForOutWhenUnconnected=off
  tag scope: onTrack=global
  wires:
  Zone collision penalty/1 -> Sum1/3, Goto1/1
  E/1 -> Sum/2
  Subsystem2/2(failCollided) -> Logical Operator1/2, E/1
  Overtaking/1(r_ot) -> Sum1/2
  B/1 -> Sum/4
  Subsystem2/4(overtakeSuccess) -> B/1
  [ry2] -> Overtaking/1(ry)
  Path following/1(r_pf) -> Sum1/1
  e2dot/1 -> Subsystem/6(e2dot)
  e1/1 -> Abs/1, Path following/2(e1), Subsystem/3(e1), Subsystem2/2(e1)
  e2/1 -> Subsystem/4(e2), Path following/3(e2), Subsystem2/3(e2)
  v_lead/1 -> Subsystem/7(v_lead)
  xgap/1 -> Subsystem/8(xgap), Subsystem2/4(xgap), Zone collision penalty/2, Overtaking/2(G)
  Subsystem/1(obs) -> obs/1
  e1dot/1 -> Subsystem/5(e1dot)
  Gain1/1 -> Sum/1
  Abs/1 -> Compare To Constant/1
  Compare To Constant/1 -> [onTrack]
  collided/1 -> Subsystem2/5(collided)
  v_ref/1 -> Subsystem/2(v_ref)
  ygap/1 -> Subsystem/9(ygap), Zone collision penalty/1
  Subsystem/2(v_err) -> Path following/1(v_err)
  steer/1 -> Path following/4(steer)
  accel/1 -> Path following/5(accel)
  Logical Operator1/1 -> isDone/1
  v_ego/1 -> Subsystem2/1(v_ego), Subsystem/1(v_ego)
  Subsystem2/1(fail) -> Logical Operator1/1, Gain1/1
  Subsystem2/3(completeCourse) -> A/1, Logical Operator1/3
  A/1 -> Sum/3
  Sum2/1 -> Reward/1
  Sum/1 -> Sum2/1
  Sum1/1 -> Integrator/1, Sum2/2
  Integrator/1 -> Scope/1

== system rewardLibrary/Obs // Reward 8-2 ==
  xgap : Inport
  ygap : Inport  Port=2
  v_lead : Inport  Port=3
  v_ego : Inport  Port=4
  v_ref : Inport  Port=5
  e1 : Inport  Port=6
  e2 : Inport  Port=7
  e1dot : Inport  Port=8
  e2dot : Inport  Port=9
  accel : Inport  Port=10
  steer : Inport  Port=11
  collided : Inport  Port=12
  Abs : Abs  SaturateOnIntegerOverflow=off
  Compare To Constant : simulink/Logic and Bit Operations/Compare To Constant  relop=<=  const=6  OutDataTypeStr=boolean
  Gain1 : Gain  Gain=20
  Gain2 : Gain  Gain=1500
  Gain3 : Gain  Gain=B
  Gain4 : Gain  Gain=3000
  Logical Operator1 : Logic  Operator=OR  Inputs=3  AllPortsSameDT=off  OutDataTypeStr=boolean
  Overtaking : Subsystem
  Path following : Subsystem
  Subsystem : Subsystem
  Subsystem2 : Subsystem
  Sum : Sum  Inputs=--++++-
  Zone collision penalty : Lookup_n-D  BreakpointsForDimension1=x_colpen  BreakpointsForDimension2=y_colpen  Table=Z_colpen  ExtrapMethod=Clip  InternalRulePriority=Speed  RndMeth=Simplest
      settings: InputPortMap=u0,u1
      mask Display:
      | image("LookupTable.PNG")
      | port_label('input', 1, 'x')
      | port_label('input', 2, 'y')
      | port_label('output', 1, 'p_col')
  obs : Outport  VectorParamsAs1DForOutWhenUnconnected=off
  Reward : Outport  Port=2  VectorParamsAs1DForOutWhenUnconnected=off
  isDone : Outport  Port=3  VectorParamsAs1DForOutWhenUnconnected=off
  tag scope: onTrack=global
  wires:
  Gain2/1 -> Sum/3
  Subsystem2/3(completeCourse) -> Logical Operator1/3, Gain2/1
  Subsystem2/1(fail) -> Gain1/1, Logical Operator1/1
  v_ego/1 -> Subsystem/1(v_ego), Subsystem2/1(v_ego)
  Logical Operator1/1 -> isDone/1
  accel/1 -> Path following/5(accel)
  steer/1 -> Path following/4(steer)
  Subsystem/2(v_err) -> Path following/1(v_err)
  ygap/1 -> Zone collision penalty/2, Subsystem/9(ygap)
  v_ref/1 -> Subsystem/2(v_ref)
  collided/1 -> Subsystem2/5(collided)
  Compare To Constant/1 -> [onTrack]
  Abs/1 -> Compare To Constant/1
  Gain1/1 -> Sum/1
  Sum/1 -> Reward/1
  e1dot/1 -> Subsystem/5(e1dot)
  Subsystem/1(obs) -> obs/1
  xgap/1 -> Zone collision penalty/1, Overtaking/2(G), Subsystem2/4(xgap), Subsystem/8(xgap)
  v_lead/1 -> Subsystem/7(v_lead)
  e2/1 -> Subsystem2/3(e2), Path following/3(e2), Subsystem/4(e2)
  e1/1 -> Subsystem2/2(e1), Subsystem/3(e1), Path following/2(e1), Abs/1
  e2dot/1 -> Subsystem/6(e2dot)
  Path following/1(r_pf) -> Sum/5
  [ry2] -> Overtaking/1(ry)
  Subsystem2/4(overtakeSuccess) -> Gain3/1
  Gain3/1 -> Sum/4
  Overtaking/1(r_ot) -> Sum/6
  Subsystem2/2(failCollided) -> Gain4/1, Logical Operator1/2
  Gain4/1 -> Sum/2
  Zone collision penalty/1 -> Sum/7

== system rewardLibrary/Obs // Reward 8-3 ==
  xgap : Inport
  ygap : Inport  Port=2
  v_lead : Inport  Port=3
  v_ego : Inport  Port=4
  v_ref : Inport  Port=5
  e1 : Inport  Port=6
  e2 : Inport  Port=7
  e1dot : Inport  Port=8
  e2dot : Inport  Port=9
  accel : Inport  Port=10
  steer : Inport  Port=11
  collided : Inport  Port=12
  Abs : Abs  SaturateOnIntegerOverflow=off
  Compare To Constant : simulink/Logic and Bit Operations/Compare To Constant  relop=<=  const=6  OutDataTypeStr=boolean
  Gain1 : Gain  Gain=20
  Gain2 : Gain  Gain=1500
  Gain3 : Gain  Gain=B
  Gain4 : Gain  Gain=3000
  Logical Operator1 : Logic  Operator=OR  Inputs=3  AllPortsSameDT=off  OutDataTypeStr=boolean
  Overtaking : Subsystem
  Path following : Subsystem
  Subsystem : Subsystem
  Subsystem2 : Subsystem
  Sum : Sum  Inputs=--++++-
  Zone collision penalty : Lookup_n-D  BreakpointsForDimension1=y_colpen  BreakpointsForDimension2=x_colpen  Table=Z_colpen  ExtrapMethod=Clip  InternalRulePriority=Speed  RndMeth=Simplest
      settings: InputPortMap=u0,u1
      mask Display:
      | image("LookupTable.PNG")
      | port_label('input', 1, 'y')
      | port_label('input', 2, 'x')
      | port_label('output', 1, 'p_col')
  obs : Outport  VectorParamsAs1DForOutWhenUnconnected=off
  Reward : Outport  Port=2  VectorParamsAs1DForOutWhenUnconnected=off
  isDone : Outport  Port=3  VectorParamsAs1DForOutWhenUnconnected=off
  tag scope: onTrack=global, p_col=global
  wires:
  Gain2/1 -> Sum/3
  Subsystem2/3(completeCourse) -> Logical Operator1/3, Gain2/1
  Subsystem2/1(fail) -> Gain1/1, Logical Operator1/1
  v_ego/1 -> Subsystem/1(v_ego), Subsystem2/1(v_ego)
  Logical Operator1/1 -> isDone/1
  accel/1 -> Path following/5(accel)
  steer/1 -> Path following/4(steer)
  Subsystem/2(v_err) -> Path following/1(v_err)
  ygap/1 -> Zone collision penalty/1, Subsystem/9(ygap)
  v_ref/1 -> Subsystem/2(v_ref)
  collided/1 -> Subsystem2/5(collided)
  Compare To Constant/1 -> [onTrack]
  Abs/1 -> Compare To Constant/1
  Gain1/1 -> Sum/1
  Sum/1 -> Reward/1
  e1dot/1 -> Subsystem/5(e1dot)
  Subsystem/1(obs) -> obs/1
  xgap/1 -> Overtaking/2(G), Zone collision penalty/2, Subsystem2/4(xgap), Subsystem/8(xgap)
  v_lead/1 -> Subsystem/7(v_lead)
  e2/1 -> Subsystem2/3(e2), Path following/3(e2), Subsystem/4(e2)
  e1/1 -> Subsystem2/2(e1), Subsystem/3(e1), Path following/2(e1), Abs/1
  e2dot/1 -> Subsystem/6(e2dot)
  Path following/1(r_pf) -> Sum/5
  [ry2] -> Overtaking/1(ry)
  Subsystem2/4(overtakeSuccess) -> Gain3/1
  Gain3/1 -> Sum/4
  Overtaking/1(r_ot) -> Sum/6
  Subsystem2/2(failCollided) -> Gain4/1, Logical Operator1/2
  Gain4/1 -> Sum/2
  Zone collision penalty/1 -> Sum/7, [p_col]

== system rewardLibrary/Obs // Reward 8-4 ==
  xgap : Inport
  ygap : Inport  Port=2
  v_lead : Inport  Port=3
  v_ego : Inport  Port=4
  v_ref : Inport  Port=5
  e1 : Inport  Port=6
  e2 : Inport  Port=7
  e1dot : Inport  Port=8
  e2dot : Inport  Port=9
  accel : Inport  Port=10
  steer : Inport  Port=11
  collided : Inport  Port=12
  Abs : Abs  SaturateOnIntegerOverflow=off
  Compare To Constant : simulink/Logic and Bit Operations/Compare To Constant  relop=<=  const=6  OutDataTypeStr=boolean
  Gain1 : Gain  Gain=20
  Gain2 : Gain  Gain=A
  Gain3 : Gain  Gain=B
  Gain4 : Gain  Gain=E
  Logical Operator1 : Logic  Operator=OR  Inputs=3  AllPortsSameDT=off  OutDataTypeStr=boolean
  Overtaking : Subsystem
  Path following : Subsystem
  Subsystem : Subsystem
  Subsystem2 : Subsystem
  Sum : Sum  Inputs=--++++-
  Zone collision penalty : Lookup_n-D  BreakpointsForDimension1=y_colpen  BreakpointsForDimension2=x_colpen  Table=Z_colpen  ExtrapMethod=Clip  InternalRulePriority=Speed  RndMeth=Simplest
      settings: InputPortMap=u0,u1
      mask Display:
      | image("LookupTable.PNG")
      | port_label('input', 1, 'y')
      | port_label('input', 2, 'x')
      | port_label('output', 1, 'p_col')
  obs : Outport  VectorParamsAs1DForOutWhenUnconnected=off
  Reward : Outport  Port=2  VectorParamsAs1DForOutWhenUnconnected=off
  isDone : Outport  Port=3  VectorParamsAs1DForOutWhenUnconnected=off
  tag scope: onTrack=global, p_col=global
  wires:
  Gain2/1 -> Sum/3
  Subsystem2/3(completeCourse) -> Logical Operator1/3, Gain2/1
  Subsystem2/1(fail) -> Gain1/1, Logical Operator1/1
  v_ego/1 -> Subsystem/1(v_ego), Subsystem2/1(v_ego)
  Logical Operator1/1 -> isDone/1
  accel/1 -> Path following/5(accel)
  steer/1 -> Path following/4(steer)
  Subsystem/2(v_err) -> Path following/1(v_err)
  ygap/1 -> Zone collision penalty/1, Subsystem/9(ygap)
  v_ref/1 -> Subsystem/2(v_ref)
  collided/1 -> Subsystem2/5(collided)
  Compare To Constant/1 -> [onTrack]
  Abs/1 -> Compare To Constant/1
  Gain1/1 -> Sum/1
  Sum/1 -> Reward/1
  e1dot/1 -> Subsystem/5(e1dot)
  Subsystem/1(obs) -> obs/1
  xgap/1 -> Overtaking/2(G), Zone collision penalty/2, Subsystem2/4(xgap), Subsystem/8(xgap)
  v_lead/1 -> Subsystem/7(v_lead)
  e2/1 -> Subsystem2/3(e2), Path following/3(e2), Subsystem/4(e2)
  e1/1 -> Subsystem2/2(e1), Subsystem/3(e1), Path following/2(e1), Abs/1
  e2dot/1 -> Subsystem/6(e2dot)
  Path following/1(r_pf) -> Sum/5
  [ry2] -> Overtaking/1(ry)
  Subsystem2/4(overtakeSuccess) -> Gain3/1
  Gain3/1 -> Sum/4
  Overtaking/1(r_ot) -> Sum/6
  Subsystem2/2(failCollided) -> Gain4/1, Logical Operator1/2
  Gain4/1 -> Sum/2
  Zone collision penalty/1 -> Sum/7, [p_col]

== system rewardLibrary/Obs // Reward 8-5 ==
  xgap : Inport
  ygap : Inport  Port=2
  v_lead : Inport  Port=3
  v_ego : Inport  Port=4
  v_ref : Inport  Port=5
  e1 : Inport  Port=6
  e2 : Inport  Port=7
  e1dot : Inport  Port=8
  e2dot : Inport  Port=9
  accel : Inport  Port=10
  steer : Inport  Port=11
  collided : Inport  Port=12
  A : Gain  Gain=A
  Abs : Abs  SaturateOnIntegerOverflow=off
  B : Gain  Gain=B
  Compare To Constant : simulink/Logic and Bit Operations/Compare To Constant  relop=<=  const=6  OutDataTypeStr=boolean
  E : Gain  Gain=E
  Gain1 : Gain  Gain=20
  Logical Operator1 : Logic  Operator=OR  Inputs=3  AllPortsSameDT=off  OutDataTypeStr=boolean
  Overtaking : Subsystem
  Path following : Subsystem
  Subsystem : Subsystem
  Subsystem2 : Subsystem
  Sum : Sum  Inputs=--+++++
  Zone collision penalty : Lookup_n-D  BreakpointsForDimension1=y_colpen  BreakpointsForDimension2=x_colpen  Table=Z_colpen  ExtrapMethod=Clip  InternalRulePriority=Speed  RndMeth=Simplest
      settings: InputPortMap=u0,u1
      mask Display:
      | image("LookupTable.PNG")
      | port_label('input', 1, 'y')
      | port_label('input', 2, 'x')
      | port_label('output', 1, 'p_col')
  obs : Outport  VectorParamsAs1DForOutWhenUnconnected=off
  Reward : Outport  Port=2  VectorParamsAs1DForOutWhenUnconnected=off
  isDone : Outport  Port=3  VectorParamsAs1DForOutWhenUnconnected=off
  tag scope: onTrack=global, p_col=global
  wires:
  A/1 -> Sum/3
  Subsystem2/3(completeCourse) -> Logical Operator1/3, A/1
  Subsystem2/1(fail) -> Gain1/1, Logical Operator1/1
  v_ego/1 -> Subsystem/1(v_ego), Subsystem2/1(v_ego)
  Logical Operator1/1 -> isDone/1
  accel/1 -> Path following/5(accel)
  steer/1 -> Path following/4(steer)
  Subsystem/2(v_err) -> Path following/1(v_err)
  ygap/1 -> Zone collision penalty/1, Subsystem/9(ygap)
  v_ref/1 -> Subsystem/2(v_ref)
  collided/1 -> Subsystem2/5(collided)
  Compare To Constant/1 -> [onTrack]
  Abs/1 -> Compare To Constant/1
  Gain1/1 -> Sum/1
  Sum/1 -> Reward/1
  e1dot/1 -> Subsystem/5(e1dot)
  Subsystem/1(obs) -> obs/1
  xgap/1 -> Overtaking/2(G), Zone collision penalty/2, Subsystem2/4(xgap), Subsystem/8(xgap)
  v_lead/1 -> Subsystem/7(v_lead)
  e2/1 -> Subsystem2/3(e2), Path following/3(e2), Subsystem/4(e2)
  e1/1 -> Subsystem2/2(e1), Subsystem/3(e1), Path following/2(e1), Abs/1
  e2dot/1 -> Subsystem/6(e2dot)
  Path following/1(r_pf) -> Sum/5
  [ry2] -> Overtaking/1(ry)
  Subsystem2/4(overtakeSuccess) -> B/1
  B/1 -> Sum/4
  Overtaking/1(r_ot) -> Sum/6
  Subsystem2/2(failCollided) -> E/1, Logical Operator1/2
  E/1 -> Sum/2
  Zone collision penalty/1 -> Sum/7, [p_col]

== system rewardLibrary/Obs // Reward 8-7 ==
  xgap : Inport
  ygap : Inport  Port=2
  v_lead : Inport  Port=3
  v_ego : Inport  Port=4
  v_ref : Inport  Port=5
  e1 : Inport  Port=6
  e2 : Inport  Port=7
  e1dot : Inport  Port=8
  e2dot : Inport  Port=9
  accel : Inport  Port=10
  steer : Inport  Port=11
  collided : Inport  Port=12
  A : Gain  Gain=500
  Abs : Abs  SaturateOnIntegerOverflow=off
  B : Gain  Gain=0
  Compare To Constant : simulink/Logic and Bit Operations/Compare To Constant  relop=<=  const=6  OutDataTypeStr=boolean
  E : Gain  Gain=2000
  Gain1 : Gain  Gain=20
  Logical Operator1 : Logic  Operator=OR  Inputs=3  AllPortsSameDT=off  OutDataTypeStr=boolean
  Overtaking : Subsystem
  Path following : Subsystem
  Subsystem : Subsystem
  Subsystem2 : Subsystem
  Sum : Sum  Inputs=--+++++
  Zone collision penalty : Lookup_n-D  BreakpointsForDimension1=y_colpen  BreakpointsForDimension2=x_colpen  Table=Z_colpen  ExtrapMethod=Clip  InternalRulePriority=Speed  RndMeth=Simplest
      settings: InputPortMap=u0,u1
      mask Display:
      | image("LookupTable.PNG")
      | port_label('input', 1, 'y')
      | port_label('input', 2, 'x')
      | port_label('output', 1, 'p_col')
  obs : Outport  VectorParamsAs1DForOutWhenUnconnected=off
  Reward : Outport  Port=2  VectorParamsAs1DForOutWhenUnconnected=off
  isDone : Outport  Port=3  VectorParamsAs1DForOutWhenUnconnected=off
  tag scope: onTrack=global, p_col=global
  wires:
  A/1 -> Sum/3
  Subsystem2/3(completeCourse) -> Logical Operator1/3, A/1
  Subsystem2/1(fail) -> Gain1/1, Logical Operator1/1
  v_ego/1 -> Subsystem/1(v_ego), Subsystem2/1(v_ego)
  Logical Operator1/1 -> isDone/1
  accel/1 -> Path following/5(accel)
  steer/1 -> Path following/4(steer)
  Subsystem/2(v_err) -> Path following/1(v_err)
  ygap/1 -> Zone collision penalty/1, Subsystem/9(ygap)
  v_ref/1 -> Subsystem/2(v_ref)
  collided/1 -> Subsystem2/5(collided)
  Compare To Constant/1 -> [onTrack]
  Abs/1 -> Compare To Constant/1
  Gain1/1 -> Sum/1
  Sum/1 -> Reward/1
  e1dot/1 -> Subsystem/5(e1dot)
  Subsystem/1(obs) -> obs/1
  xgap/1 -> Overtaking/2(G), Zone collision penalty/2, Subsystem2/4(xgap), Subsystem/8(xgap)
  v_lead/1 -> Subsystem/7(v_lead)
  e2/1 -> Subsystem2/3(e2), Path following/3(e2), Subsystem/4(e2)
  e1/1 -> Subsystem2/2(e1), Subsystem/3(e1), Path following/2(e1), Abs/1
  e2dot/1 -> Subsystem/6(e2dot)
  Path following/1(r_pf) -> Sum/5
  [ry2] -> Overtaking/1(ry)
  Subsystem2/4(overtakeSuccess) -> B/1
  B/1 -> Sum/4
  Overtaking/1(r_ot) -> Sum/6
  Subsystem2/2(failCollided) -> E/1, Logical Operator1/2
  E/1 -> Sum/2
  Zone collision penalty/1 -> Sum/7, [p_col]
